simulink model "Time_delay_system_tau_d_large"  (Simulink 7.6)
settings: Solver=ode45  StartTime=0.0  StopTime=10.0  RelTol=1e-3
settings Model: Creator=administrator  LastModifiedBy=administrator

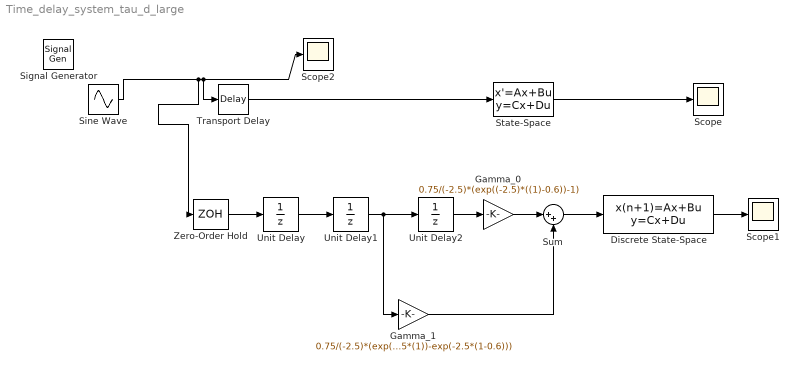
== system Time_delay_system_tau_d_large ==
  Discrete State-Space : DiscreteStateSpace  A=expm(-2.5*1)  D=0  SampleTime=-1
  Gamma_0 : Gain  Gain=0.75/(-2.5)*(exp((-2.5)*((1)-0.6))-1)
  Gamma_1 : Gain  Gain=0.75/(-2.5)*(exp(-2.5*(1))-exp(-2.5*(1-0.6)))
  Scope : Scope
      settings: TickLabels=on  TimeRange=10
  Scope1 : Scope
      settings: TickLabels=on  TimeRange=10
  Scope2 : Scope
      settings: SaveName=ScopeData2
  Signal Generator : SignalGenerator  WaveForm=square  Frequency=pi  Units=rad/sec
  Sine Wave : Sin  SampleTime=0
  State-Space : StateSpace  A=-2.5  B=0.75  D=0
  Sum : Sum  Inputs=|++
  Transport Delay : TransportDelay  DelayTime=3
  Unit Delay : UnitDelay  SampleTime=-1
  Unit Delay1 : UnitDelay  SampleTime=-1
  Unit Delay2 : UnitDelay  SampleTime=-1
  Zero-Order Hold : ZeroOrderHold
  wires:
  Transport Delay/1 -> State-Space/1
  State-Space/1 -> Scope/1
  Zero-Order Hold/1 -> Unit Delay/1
  Sum/1 -> Discrete State-Space/1
  Discrete State-Space/1 -> Scope1/1
  Unit Delay/1 -> Unit Delay1/1
  Unit Delay1/1 -> Unit Delay2/1, Gamma_1/1
  Unit Delay2/1 -> Gamma_0/1
  Gamma_1/1 -> Sum/2
  Gamma_0/1 -> Sum/1
  Sine Wave/1 -> Zero-Order Hold/1, Scope2/1, Transport Delay/1
